simulink model "testStateflow"  (R2015b)
settings: Solver=VariableStepAuto  StartTime=0.0  StopTime=10.0  RelTol=1e-3
settings Model: Creator=barbot  LastModifiedBy=barbot

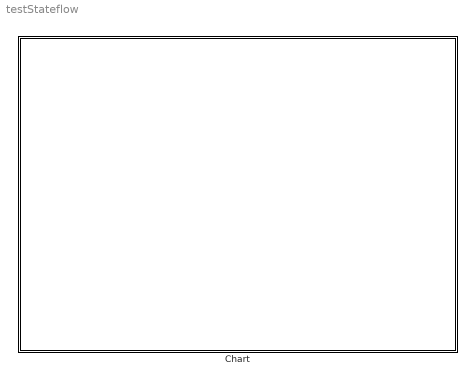
== system testStateflow ==
  Chart : Stateflow chart  TreatAsAtomicUnit=on

== stateflow chart testStateflow/Chart ==
  state Main
    state A1 [parallel]
      settings: executionOrder=1
      state On
      state Off
      Main.A1.On -> Main.A1.Off : after(1,msec)
      (default) -> Main.A1.On
      Main.A1.Off -> Main.A1.On : after(2,msec)
    state A2 [parallel]
      settings: executionOrder=2
      state On
      state Off
      Main.A2.On -> Main.A2.Off : after(1,msec)
      (default) -> Main.A2.On
      Main.A2.Off -> Main.A2.On : after(2,msec)
